simulink subsystem "rocket"  (R2024b)
settings: Solver=VariableStepAuto  StartTime=0.0  StopTime=10.0  RelTol=1e-3
undefined symbols (not defined in the file or in its folder): airdata, GRAVITY, GROUND_LEVEL, MASS_DRY, plate_area, plate_num, position_init, REF_AREA, use_custom_atm, velocity_init
libraries: aerolibatmos2 x1
settings Model: Creator=yevge  LastModifiedBy=Aiden Gaydos

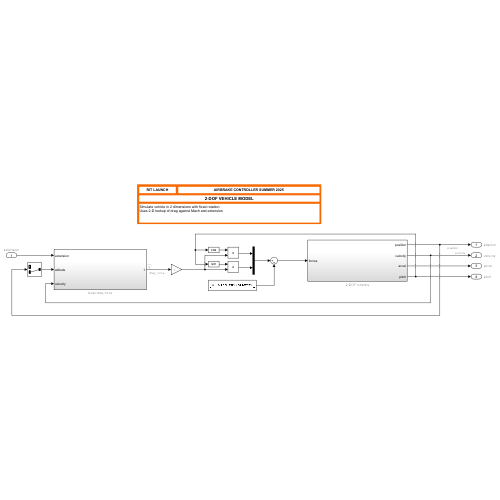
[thumbnail: Simulink's stored preview of the top-level diagram]
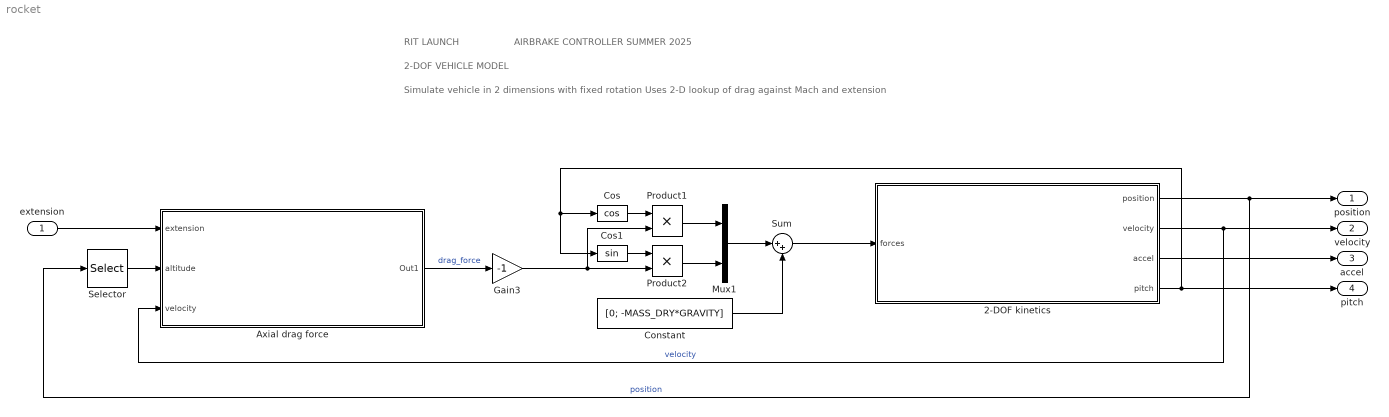
== system rocket ==
  note: RIT LAUNCH
  note: AIRBRAKE CONTROLLER SUMMER 2025
  note: Simulate vehicle in 2 dimensions with fixed rotation
      | Uses 2-D lookup of drag against Mach and extension
  note: 2-DOF VEHICLE MODEL
  extension : Inport  OutMin=0  OutMax=1  Unit=1  PortDimensions=1
  2-DOF kinetics : Subsystem
  Axial drag force : Subsystem
  Constant : Constant  Value=[0; -MASS_DRY*GRAVITY]
  Cos : Trigonometry  Operator=cos
  Cos1 : Trigonometry
  Gain3 : Gain  Gain=-1
  Mux1 : Mux  Inputs=2
  Product1 : Product
  Product2 : Product
  Selector : Selector  InputPortWidth=2  IndexOptions=Index vector (dialog)  Indices=2  OutputSizes=1
  Sum : Sum  Inputs=|++
  position : Outport  Unit=m  PortDimensions=[2 1]
  velocity : Outport  Port=2  Unit=m/s  PortDimensions=[2 1]
  accel : Outport  Port=3  Unit=m/s^2  PortDimensions=[2 1]
  pitch : Outport  Port=4  Unit=rad  PortDimensions=1
  wires:
  Product1/1 -> Mux1/1
  Constant/1 -> Sum/2
  Sum/1 -> 2-DOF kinetics/1(forces)
  Product2/1 -> Mux1/2
  Gain3/1 -> Product2/2, Product1/2
  Cos1/1 -> Product2/1
  2-DOF kinetics/4(pitch) -> Cos/1, Cos1/1, pitch/1
  Cos/1 -> Product1/1
  Mux1/1 -> Sum/1
  Axial drag force/1(Out1) -> Gain3/1  "drag_force"
  2-DOF kinetics/2(velocity) -> Axial drag force/3(velocity), velocity/1  "velocity"
  2-DOF kinetics/1(position) -> Selector/1, position/1  "position"
  2-DOF kinetics/3(accel) -> accel/1
  extension/1 -> Axial drag force/1(extension)
  Selector/1 -> Axial drag force/2(altitude)

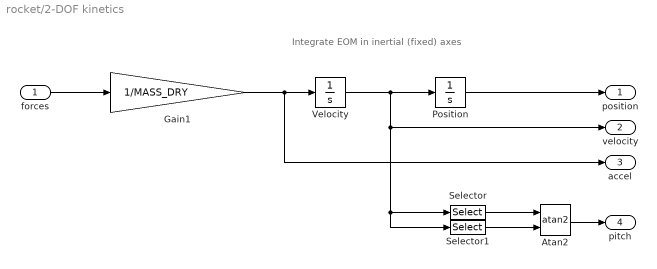
== system rocket/2-DOF kinetics ==
  note: Integrate EOM in inertial (fixed) axes
  forces : Inport  Unit=N  PortDimensions=[2 1]
  Atan2 : Trigonometry  Operator=atan2
  Gain1 : Gain  Gain=1/MASS_DRY
  Position : Integrator  InitialCondition=position_init  ContinuousStateAttributes='position'
  Selector : Selector  InputPortWidth=2  IndexOptions=Index vector (dialog)  Indices=2  OutputSizes=1
  Selector1 : Selector  InputPortWidth=2  IndexOptions=Index vector (dialog)  Indices=1  OutputSizes=1
  Velocity : Integrator  InitialCondition=velocity_init  ContinuousStateAttributes='velocity'
  position : Outport  Unit=m  PortDimensions=[2 1]
  velocity : Outport  Port=2  Unit=m/s  PortDimensions=[2 1]
  accel : Outport  Port=3  Unit=m/s^2  PortDimensions=[2 1]
  pitch : Outport  Port=4  Unit=rad  PortDimensions=1
  wires:
  Atan2/1 -> pitch/1
  Selector1/1 -> Atan2/2
  Selector/1 -> Atan2/1
  Position/1 -> position/1
  forces/1 -> Gain1/1
  Gain1/1 -> Velocity/1, accel/1
  Velocity/1 -> Position/1, velocity/1, Selector/1, Selector1/1

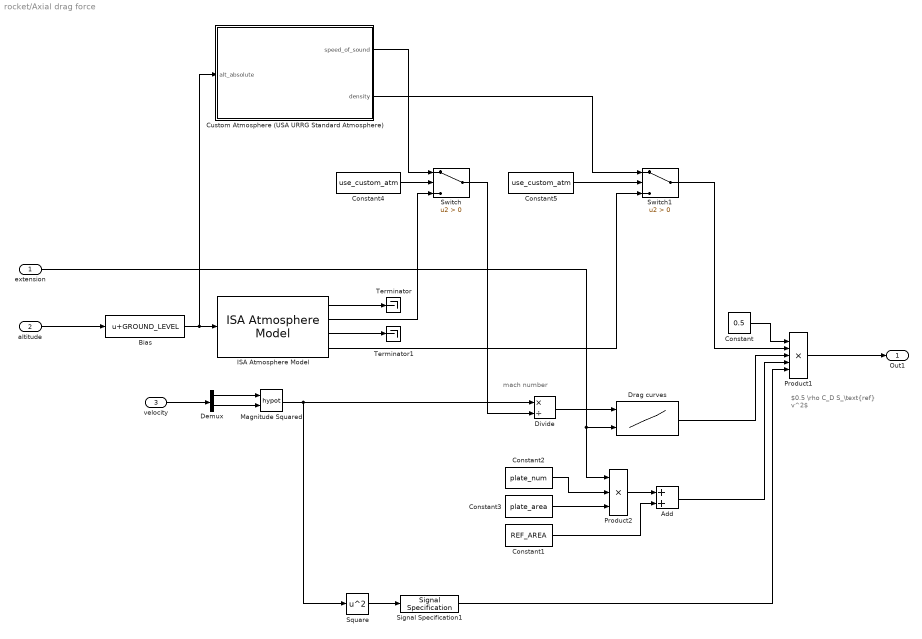
== system rocket/Axial drag force ==
  note: $0.5 \rho C_D S_\text{ref} v^2$
  note: mach number
  extension : Inport  OutMin=0  OutMax=1  Unit=1  PortDimensions=1
  altitude : Inport  Port=2  Unit=m  PortDimensions=1
  velocity : Inport  Port=3  Unit=m/s  PortDimensions=[2 1]
  Add : Sum
  Bias : Bias  Bias=GROUND_LEVEL  SaturateOnIntegerOverflow=off
  Constant : Constant  Value=0.5
  Constant1 : Constant  Value=REF_AREA
  Constant2 : Constant  Value=plate_num
  Constant3 : Constant  Value=plate_area
  Constant4 : Constant  Value=use_custom_atm
  Constant5 : Constant  Value=use_custom_atm
  Custom Atmosphere (USA URRG Standard Atmosphere) : Subsystem
  Demux : Demux  Outputs=2
  Divide : Product  Inputs=*/
  Drag curves : Lookup_n-D  DataSpecification=Lookup table object  LookupTableObject=DRAG_LUT  BreakpointsForDimension1=[1:3]  BreakpointsForDimension2=[1:3]  InternalRulePriority=Speed  RndMeth=Simplest
      settings: InputPortMap=u0,u1
  ISA Atmosphere Model : aerolibatmos2/ISA Atmosphere Model  useExtended=off  action=Warning  custom=off  viscosityOut=off  g=9.80665  gamma=1.4  R=287.0531  L=0.0065  h_trop=11000  h_strat=20000  rho0=1.225  P0=101325  T0=288.15  h0=0  S=110.4  Tref=273.15  muref=1.716e-5
  Magnitude Squared : Math  Operator=hypot
  Product1 : Product  Inputs=5
  Product2 : Product  Inputs=3
  Signal Specification1 : SignalSpecification  Unit=m^2/s^2  Dimensions=1
  Square : Math  Operator=square
  Switch : Switch  Criteria=u2 > Threshold  SaturateOnIntegerOverflow=off  InputSameDT=off
  Switch1 : Switch  Criteria=u2 > Threshold  SaturateOnIntegerOverflow=off  InputSameDT=off
  Terminator : Terminator
  Terminator1 : Terminator
  Out1 : Outport  Unit=N  PortDimensions=1
  wires:
  Constant5/1 -> Switch1/2
  Custom Atmosphere (USA URRG Standard Atmosphere)/2(density) -> Switch1/1
  Switch1/1 -> Product1/2
  Constant4/1 -> Switch/2
  Switch/1 -> Divide/2
  Custom Atmosphere (USA URRG Standard Atmosphere)/1(speed_of_sound) -> Switch/1
  ISA Atmosphere Model/2 -> Switch/3
  Signal Specification1/1 -> Product1/5
  Drag curves/1 -> Product1/3
  extension/1 -> Product2/1, Drag curves/2
  Divide/1 -> Drag curves/1
  Constant/1 -> Product1/1
  Square/1 -> Signal Specification1/1
  ISA Atmosphere Model/3 -> Terminator1/1
  ISA Atmosphere Model/1 -> Terminator/1
  Magnitude Squared/1 -> Divide/1, Square/1
  Demux/2 -> Magnitude Squared/2
  Demux/1 -> Magnitude Squared/1
  Bias/1 -> ISA Atmosphere Model/1, Custom Atmosphere (USA URRG Standard Atmosphere)/1(alt_absolute)
  altitude/1 -> Bias/1
  Product1/1 -> Out1/1
  velocity/1 -> Demux/1
  Constant3/1 -> Product2/3
  Constant2/1 -> Product2/2
  Constant1/1 -> Add/2
  Product2/1 -> Add/1
  Add/1 -> Product1/4
  ISA Atmosphere Model/4 -> Switch1/3

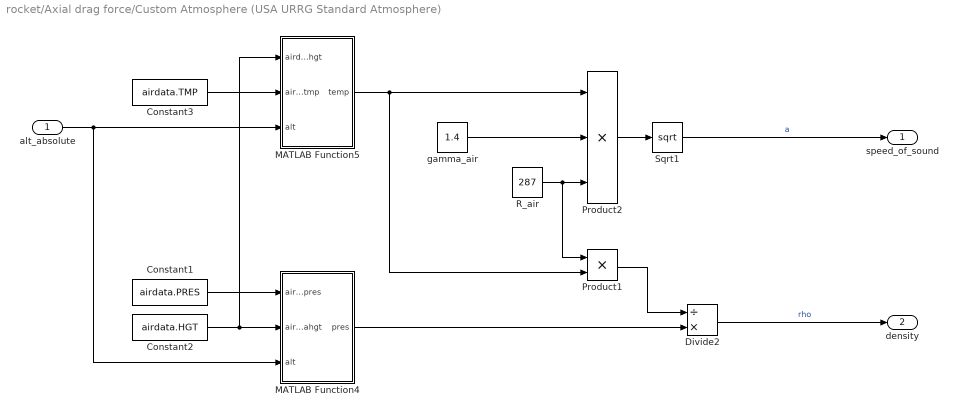
== system rocket/Axial drag force/Custom Atmosphere (USA URRG Standard Atmosphere) ==
  alt_absolute : Inport
  Constant1 : Constant  Value=airdata.PRES
  Constant2 : Constant  Value=airdata.HGT
  Constant3 : Constant  Value=airdata.TMP
  Divide2 : Product  Inputs=/*
  MATLAB Function4 : MATLAB Function  TreatAsAtomicUnit=on
  MATLAB Function5 : MATLAB Function  TreatAsAtomicUnit=on
  Product1 : Product
  Product2 : Product  Inputs=3
  R_air : Constant  Value=287
  Sqrt1 : Sqrt
  gamma_air : Constant  Value=1.4
  speed_of_sound : Outport
  density : Outport  Port=2
  wires:
  Constant3/1 -> MATLAB Function5/2(airdatatmp)
  Constant2/1 -> MATLAB Function4/2(airdatahgt), MATLAB Function5/1(airdatahgt)
  Divide2/1 -> density/1  "rho"
  MATLAB Function4/1(pres) -> Divide2/2
  Product1/1 -> Divide2/1
  gamma_air/1 -> Product2/2
  R_air/1 -> Product2/3, Product1/1
  MATLAB Function5/1(temp) -> Product2/1, Product1/2
  Sqrt1/1 -> speed_of_sound/1  "a"
  alt_absolute/1 -> MATLAB Function5/3(alt), MATLAB Function4/3(alt)
  Product2/1 -> Sqrt1/1
  Constant1/1 -> MATLAB Function4/1(airdatapres)

== matlab function rocket/Axial drag force/Custom Atmosphere (USA URRG Standard Atmosphere)/MATLAB Function4 ==
  data: airdatapres input; airdatahgt input; alt input; pres output
function pres = alt_to_pres(airdatapres,airdatahgt,alt)
    pres = double(interp1(airdatahgt,airdatapres,alt,"linear","extrap"));
end

== matlab function rocket/Axial drag force/Custom Atmosphere (USA URRG Standard Atmosphere)/MATLAB Function5 ==
  data: airdatahgt input; airdatatmp input; alt input; temp output
function temp = alt_to_temp(airdatahgt,airdatatmp,alt)
    temp = double(interp1(airdatahgt,airdatatmp,alt,"linear","extrap"));
end
